simulink model "Simplus_Dual_Manual"  (R2022b)
settings: Solver=ode3  StartTime=0.0  StopTime=inf  FixedStep=Ts  RelTol=1e-3  EnableMultiTasking=on
InitFcn:
  | Ts = 100e-6;
model workspace (MAT data in the model file):
  Fbase = 50
  Filter_Ind = 0.00435
  Shunt_C = 2.2e-06
  Test_Interval = 5
  Ts = 0.0001
  VDCref = 48
undefined symbols (not defined in the file): DiscIntNeverNeededParam
libraries: rtpi x45, spsabctodq0Lib x4, spsdq0toabcLib x2, simulink x1
(part 2 of 2)

== system Simplus_Dual_Manual/GFM Inverter/Voltage Controller/PI ==
  e : Inport
  RST : Inport  Port=2
  Discrete-Time Integrator : DiscreteIntegrator  gainval=1  ExternalReset=either  SampleTime=Ts  LimitOutput=on  UpperSaturationLimit=V_IntSat  LowerSaturationLimit=-V_IntSat  ICPrevOutput=DiscIntNeverNeededParam  ICPrevScaledInput=DiscIntNeverNeededParam
  Ki : Gain  Gain=Vd_Integral  SaturateOnIntegerOverflow=on  OutDataTypeStr=Inherit: Same as input  ParamDataTypeStr=Inherit: Same as input
  Kp : Gain  Gain=Vd_Proportional  SaturateOnIntegerOverflow=on  OutDataTypeStr=Inherit: Same as input  ParamDataTypeStr=Inherit: Same as input
  Sum4 : Sum  SaturateOnIntegerOverflow=on
  Out : Outport
  tag scope: GFM_Vd_Int_Out=global, GFM_Vd_PI_Out=global
  wires:
  Ki/1 -> Discrete-Time Integrator/1
  Kp/1 -> Sum4/1
  e/1 -> Ki/1, Kp/1
  Discrete-Time Integrator/1 -> [GFM_Vd_Int_Out], Sum4/2
  Sum4/1 -> [GFM_Vd_PI_Out], Out/1
  RST/1 -> Discrete-Time Integrator/2

== system Simplus_Dual_Manual/GFM Inverter/Voltage Controller/PI1 ==
  e : Inport
  RST : Inport  Port=2
  Discrete-Time Integrator : DiscreteIntegrator  gainval=1  ExternalReset=either  SampleTime=Ts  LimitOutput=on  UpperSaturationLimit=V_IntSat  LowerSaturationLimit=-V_IntSat  ICPrevOutput=DiscIntNeverNeededParam  ICPrevScaledInput=DiscIntNeverNeededParam
  Ki : Gain  Gain=Vd_Integral  SaturateOnIntegerOverflow=on  OutDataTypeStr=Inherit: Same as input  ParamDataTypeStr=Inherit: Same as input
  Kp : Gain  Gain=Vd_Proportional  SaturateOnIntegerOverflow=on  OutDataTypeStr=Inherit: Same as input  ParamDataTypeStr=Inherit: Same as input
  Sum4 : Sum  SaturateOnIntegerOverflow=on
  Out : Outport
  tag scope: GFM_Vq_Int_Out=global, GFM_Vq_PI_Out=global
  wires:
  Ki/1 -> Discrete-Time Integrator/1
  Kp/1 -> Sum4/1
  e/1 -> Ki/1, Kp/1
  RST/1 -> Discrete-Time Integrator/2
  Discrete-Time Integrator/1 -> [GFM_Vq_Int_Out], Sum4/2
  Sum4/1 -> [GFM_Vq_PI_Out], Out/1
